simulink model "shaping"  (R2015a)
settings: Solver=ode3  StartTime=0.0  StopTime=10.0  FixedStep=1/200  RelTol=1e-3
undefined symbols (not defined in the file): gain, pole1, zero1, zero2
libraries: PoliArd x6, simulink x4
settings Model: ExtModeTrigDuration=2  Creator=GSavaia  LastModifiedBy=GSavaia
settings OptimizationCC: OptimizeModelRefInitCode=on  LifeSpan=1
settings DebuggingCC: UnderspecifiedInitializationDetection=Classic  MergeDetectMultiDrivingBlocksExec=none
settings HardwareCC: ProdLargestAtomicInteger=Long  ProdLargestAtomicFloat=Double  ProdEndianess=LittleEndian  ProdHWDeviceType=ARM Compatible->ARM Cortex
settings RTWCC: SystemTargetFile=realtime.tlc  GenerateMakefile=off  TemplateMakefile=realtime.tmf  Description=Run on Target Hardware  RTWVerbose=off
settings ERTTargetCC: CombineOutputUpdateFcns=off  ExtModeTransport=3  ExtModeMexFile=ext_serial_win32_comm_rtt  ExtModeMexArgs=0 1 9600  ERTSrcFileBannerTemplate=realtime_code_template.cgt  ERTHdrFileBannerTemplate=realtime_code_template.cgt  ERTDataSrcFileTemplate=realtime_code_template.cgt  ERTDataHdrFileTemplate=realtime_code_template.cgt  ERTCustomFileTemplate=realtime_file_process.tlc

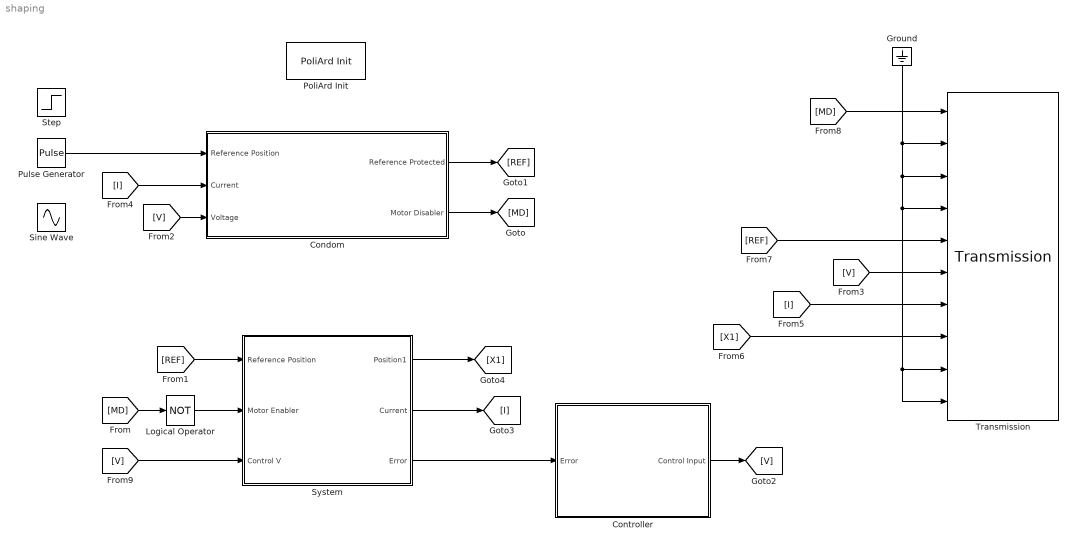
== system shaping ==
  Condom : Subsystem
  Controller : Subsystem
  Ground : Ground
  Logical Operator : Logic  Operator=NOT  AllPortsSameDT=off  OutDataTypeStr=boolean
  PoliArd Init : PoliArd/PoliArd Init
  Pulse Generator : DiscretePulseGenerator  PulseType=Time based  Period=5  PulseWidth=50
  Sine Wave : Sin  Amplitude=2  SampleTime=0
  Step : Step  SampleTime=0
  "System " : Subsystem
  Transmission : PoliArd/Transmission  sample_freq=200  sig_to_send=6
  wires:
  Ground/1 -> Transmission/3, Transmission/10, Transmission/9, Transmission/4, Transmission/2
  Logical Operator/1 -> "System "/2(Motor Enabler)
  Pulse Generator/1 -> Condom/1(Reference Position)
  Condom/2(Motor Disabler) -> [MD]
  [MD] -> Logical Operator/1
  Condom/1(Reference Protected) -> [REF]
  [REF] -> "System "/1(Reference Position)
  Controller/1(Control Input) -> [V]
  "System "/2(Current) -> [I]
  [V] -> Condom/3(Voltage)
  [V] -> Transmission/6
  [I] -> Condom/2("Current ")
  [I] -> Transmission/7
  "System "/1(Position1) -> [X1]
  [X1] -> Transmission/8
  [REF] -> Transmission/5
  [MD] -> Transmission/1
  [V] -> "System "/3(Control V)
  "System "/3(Error) -> Controller/1(Error)

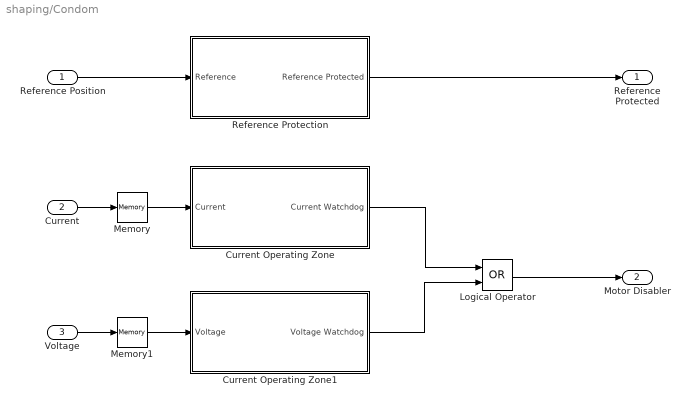
== system shaping/Condom ==
  Reference Position : Inport
  "Current " : Inport  Port=2
  Voltage : Inport  Port=3
  Current Operating Zone : Subsystem
  Current Operating Zone1 : Subsystem
  Logical Operator : Logic  Operator=OR  AllPortsSameDT=off  OutDataTypeStr=boolean
  Memory : Memory
  Memory1 : Memory
  Reference Protection : Subsystem
  Reference Protected : Outport
  Motor Disabler : Outport  Port=2
  wires:
  Current Operating Zone1/1(Voltage Watchdog) -> Logical Operator/2
  Current Operating Zone/1(Current Watchdog) -> Logical Operator/1
  Logical Operator/1 -> Motor Disabler/1
  Reference Position/1 -> Reference Protection/1("Reference ")
  Reference Protection/1(Reference Protected) -> Reference Protected/1
  Memory/1 -> Current Operating Zone/1(Current)
  "Current "/1 -> Memory/1
  Memory1/1 -> Current Operating Zone1/1(Voltage)
  Voltage/1 -> Memory1/1

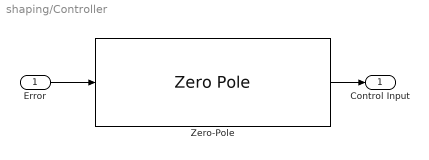
== system shaping/Controller ==
  Error : Inport
  Zero-Pole : ZeroPole  Zeros=[zero1, zero2]  Poles=[0, pole1]  Gain=gain
  Control Input : Outport
  wires:
  Zero-Pole/1 -> Control Input/1
  Error/1 -> Zero-Pole/1

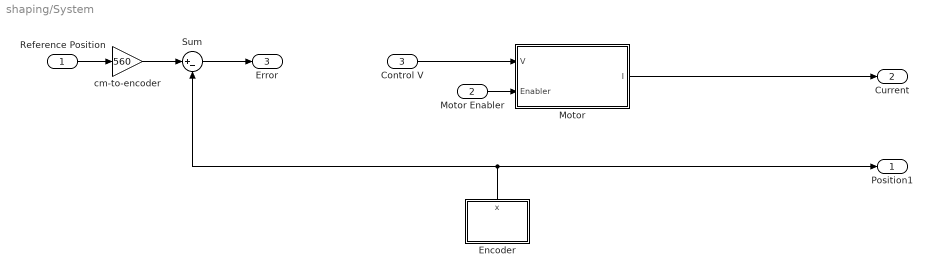
== system shaping/System  ==
  Reference Position : Inport
  Motor Enabler : Inport  Port=2
  Control V : Inport  Port=3
  "Encoder " : Subsystem
  Motor : Subsystem
  Sum : Sum  Inputs=|+-
  cm-to-encoder : Gain  Gain=560
  Position1 : Outport
  Current : Outport  Port=2
  Error : Outport  Port=3
  wires:
  "Encoder "/1(x) -> Position1/1, Sum/2
  cm-to-encoder/1 -> Sum/1
  Motor/1(I) -> Current/1
  Sum/1 -> Error/1
  Reference Position/1 -> cm-to-encoder/1
  Motor Enabler/1 -> Motor/2(Enabler)
  Control V/1 -> Motor/1(V)

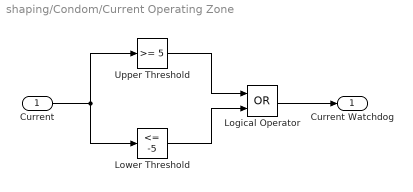
== system shaping/Condom/Current Operating Zone ==
  Current : Inport
  Logical Operator : Logic  Operator=OR  AllPortsSameDT=off  OutDataTypeStr=boolean
  Lower Threshold : simulink/Logic and Bit Operations/Compare To Constant  relop=<=  const=-5  OutDataTypeStr=boolean
  Upper Threshold : simulink/Logic and Bit Operations/Compare To Constant  relop=>=  const=5  OutDataTypeStr=boolean
  Current Watchdog : Outport
  wires:
  Lower Threshold/1 -> Logical Operator/2
  Upper Threshold/1 -> Logical Operator/1
  Logical Operator/1 -> Current Watchdog/1
  Current/1 -> Upper Threshold/1, Lower Threshold/1

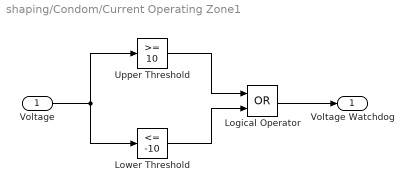
== system shaping/Condom/Current Operating Zone1 ==
  Voltage : Inport
  Logical Operator : Logic  Operator=OR  AllPortsSameDT=off  OutDataTypeStr=boolean
  Lower Threshold : simulink/Logic and Bit Operations/Compare To Constant  relop=<=  const=-10  OutDataTypeStr=boolean
  Upper Threshold : simulink/Logic and Bit Operations/Compare To Constant  relop=>=  const=10  OutDataTypeStr=boolean
  Voltage Watchdog : Outport
  wires:
  Lower Threshold/1 -> Logical Operator/2
  Upper Threshold/1 -> Logical Operator/1
  Logical Operator/1 -> Voltage Watchdog/1
  Voltage/1 -> Upper Threshold/1, Lower Threshold/1

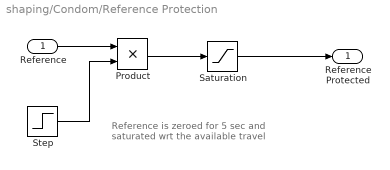
== system shaping/Condom/Reference Protection ==
  note: Reference is zeroed for 5 sec
      | and saturated wrt the available travel
  "Reference " : Inport
  Product : Product
  Saturation : Saturate  UpperLimit=3  LowerLimit=-3
  Step : Step  Time=5  SampleTime=0
  Reference Protected : Outport
  wires:
  Saturation/1 -> Reference Protected/1
  Product/1 -> Saturation/1
  "Reference "/1 -> Product/1
  Step/1 -> Product/2

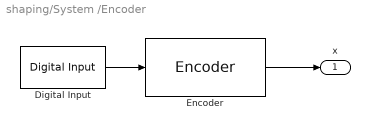
== system shaping/System /Encoder  ==
  Digital Input : PoliArd/Digital Input  DI_pin=2  DIsample=1/200
  Encoder : PoliArd/Encoder  EncoderID=1  dt_enc=1/200
  x : Outport
  wires:
  Digital Input/1 -> Encoder/1
  Encoder/1 -> x/1

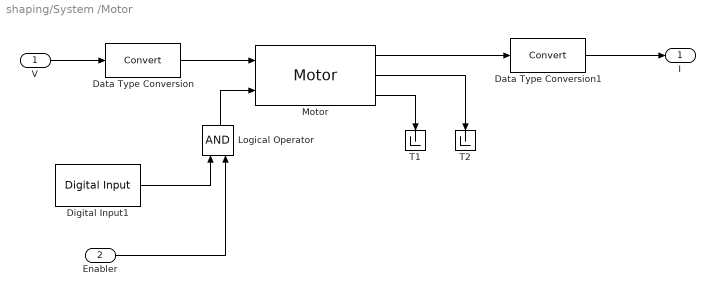
== system shaping/System /Motor ==
  V : Inport
  Enabler : Inport  Port=2
  Data Type Conversion : DataTypeConversion
  Data Type Conversion1 : DataTypeConversion
  Digital Input1 : PoliArd/Digital Input  DI_pin=3  DIsample=1/200
  Logical Operator : Logic  AllPortsSameDT=off  OutDataTypeStr=boolean
  Motor : PoliArd/Motor  MotorID=2  DC_bus_mask=12  dt_mot=1/200
  T1 : Terminator
  T2 : Terminator
  I : Outport
  wires:
  Data Type Conversion/1 -> Motor/1
  V/1 -> Data Type Conversion/1
  Motor/3 -> T1/1
  Motor/2 -> T2/1
  Motor/1 -> Data Type Conversion1/1
  Data Type Conversion1/1 -> I/1
  Enabler/1 -> Logical Operator/2
  Logical Operator/1 -> Motor/2
  Digital Input1/1 -> Logical Operator/1
